simulink model "Bungee_Jumper"  (R2024b)
settings: Solver=VariableStepAuto  StartTime=0.0  StopTime=100  RelTol=1e-3
settings Model: Creator=rares  LastModifiedBy=rares

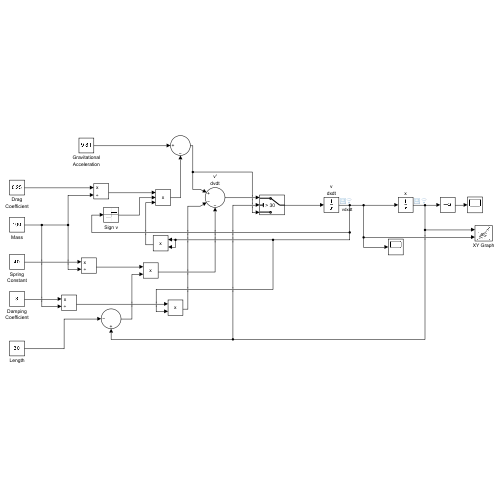
[thumbnail: Simulink's stored preview of the top-level diagram]
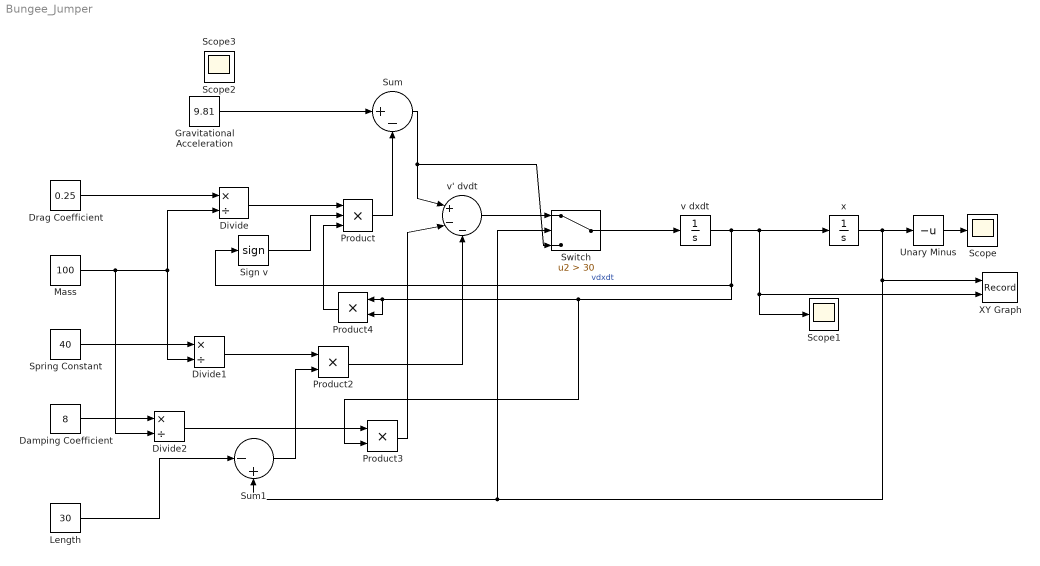
== system Bungee_Jumper ==
  Damping Coefficient : Constant  Value=8
  Divide : Product  Inputs=*/
  Divide1 : Product  Inputs=*/
  Divide2 : Product  Inputs=*/
  Drag Coefficient : Constant  Value=0.25
  Gravitational Acceleration : Constant  Value=9.81
  Length : Constant  Value=30
  Mass : Constant  Value=100
  Product : Product  Inputs=3
  Product2 : Product
  Product3 : Product
  Product4 : Product
  Scope{,1..3} (4 alike) : Scope
  Sign v : Signum
  Spring Constant : Constant  Value=40
  Sum : Sum  Inputs=|+-
  Sum1 : Sum  Inputs=|-+
  Switch : Switch  Criteria=u2 > Threshold  Threshold=30  SaturateOnIntegerOverflow=off  InputSameDT=off
  Unary Minus : UnaryMinus
  XY Graph : Record  FileSettingsInternal="{\"entries\":[{\"content\":{\"excelSettings\":{\"content\":{},\"type\":\"Streamout.ExcelSettings\"}},\"type\":\"Streamout.FileSettingStorage\",\"uuid\":\"\"}],\"packageUris\":[\"http:\\/\\/schema.mathworks.com\\/mf0\\/streamout_blocks\\/R2020a\"],\"version\":\"1.0\"}"  Layout=[1 1]  SignalsInternal="{\"entries\":[{\"content\":{\"signals\":[{\"content\":{\"blockPath\":[],\"dimensions\":[1],\"domain\":\"\",\"lineColor\":\"#a2142f\",\"plots\":[ 1 ],\"port\":1,\"sid\":[\"\"],\"signalID\":1,\"signalName\":\"x\"},\"type\":\"RecordBlkView.Signal\",\"uuid\":\"\"},{\"content\":{\"blockPath\":[],\"dimensions\":[1],\"domain\":\"\",\"lineColor\":\"#139fff\",\"plots\":[ 1 ],\"port\":2,\"sid\":[\"\"],\"signalID\":2,\"signalName\":\"vdxdt\"},\"type\":\"RecordBlkView.Signal\",\"uuid\":\"\"}]},\"type\":\"RecordBlkView.InputSignals\",\"uuid\":\"\"}],\"packageUris\":[\"http:\\/\\/schema.mathworks.com\\/mf0\\/streamout_blocks\\/R2020a\"],\"version\":\"1.0\"}"  VisualizationBindings="{\"xyplotplugin\":{\"info\":[{\"series\":[{\"bindingParametersList\":[{\"parameter\":\"X-Axis\",\"signalID\":1,\"signalName\":\"x\"},{\"parameter\":\"Y-Axis\",\"signalID\":2,\"signalName\":\"vdxdt\"}],\"seriesID\":0}],\"subplotID\":1}]}}"  CompatibilityTag=XY
  v dxdt : Integrator
  v' dvdt : Sum  Inputs=|+--
  x : Integrator
  wires:
  Drag Coefficient/1 -> Divide/1
  Mass/1 -> Divide2/2, Divide1/2, Divide/2
  Divide/1 -> Product/1
  Spring Constant/1 -> Divide1/1
  Divide1/1 -> Product2/1
  Sum1/1 -> Product2/2
  Product2/1 -> v' dvdt/3
  Damping Coefficient/1 -> Divide2/1
  Divide2/1 -> Product3/1
  Product3/1 -> v' dvdt/2
  v dxdt/1 -> XY Graph/2, Scope1/1, x/1, Product3/2, Product4/2, Product4/1, Sign v/1  "vdxdt"
  Product4/1 -> Product/3
  Sign v/1 -> Product/2
  Length/1 -> Sum1/1
  x/1 -> Unary Minus/1, XY Graph/1, Switch/2, Sum1/2
  v' dvdt/1 -> Switch/1
  Switch/1 -> v dxdt/1
  Gravitational Acceleration/1 -> Sum/1
  Product/1 -> Sum/2
  Sum/1 -> v' dvdt/1, Switch/3
  Unary Minus/1 -> Scope/1
